simulink model "sysModel"  (R2017a)
settings: Solver=FixedStepDiscrete  StartTime=0.0  StopTime=10.0  FixedStep=0.1  RelTol=1e-3  EnableMultiTasking=on
settings Model: Creator=plima  LastModifiedBy=plima
settings SolverCC: AutoInsertRateTranBlk=on
settings DataIOCC: LimitDataPoints=on
settings OptimizationCC: LifeSpan=inf
settings DebuggingCC: AllowSymbolicDim=off  SFUnexpectedBacktrackingDiag=warning  SFNoUnconditionalDefaultTransitionDiag=warning  SFExecutionAtInitializationDiag=none
settings GRTTargetCC: TargetLangStandard=C89/C90 (ANSI)  GeneratePreprocessorConditionals=Disable all
settings ConfigComp: CovMetricSettings=dw  CovHtmlReporting=on  CovSaveCumulativeToWorkspaceVar=on  CovSaveSingleToWorkspaceVar=on  CovShowResultsExplorer=off  CovExternalEMLEnable=off  CovSFcnEnable=off

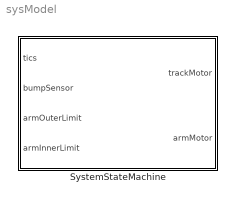
== system sysModel ==
  SystemStateMachine : Stateflow chart  TreatAsAtomicUnit=on

== stateflow chart sysModel/SystemStateMachine ==
  state ExtendArms
    entry: loopTics = tics;
    trackMotor = 0;
    during: armMotor = 1;
  state MoveOverBump
    during: armMotor = 0;
    trackMotor = 1;
  state RetractArms
    during: armMotor = -1;
  state BumpRetractArms
    during: armMotor = -1
  state MoveForward
    during: armMotor = 0;
    trackMotor = 1;
  state BumpExtendArms
    entry: loopTics = tics;
    trackMotor = 0;
    during: armMotor = 1
  state SystemStop
    during: armMotor = 0;
  state FinalRetractArms
    during: armMotor = -1;
  state FinalExtendArms
    entry: trackMotor = 0;
    during: armMotor = 1;
  (default) -> ExtendArms : /{initialTics = tics}
  MoveOverBump -> ExtendArms : [tics - loopTics >= VehicleLength + BumpLength]
  MoveForward -> ExtendArms [order 1] : [tics - loopTics >= VehicleLength]
  BumpRetractArms -> MoveOverBump : [armInnerLimit == 1]
  ExtendArms -> RetractArms : [armOuterLimit == 1]
  BumpExtendArms -> BumpRetractArms : [armOuterLimit == 1]
  RetractArms -> MoveForward : [armInnerLimit == 1]
  MoveForward -> BumpExtendArms [order 2] : [bumpSensor == 1]
  MoveForward -> FinalExtendArms [order 3] : [tics >= WindowLength + initialTics]
  FinalRetractArms -> SystemStop : [armInnerLimit == 1]
  FinalExtendArms -> FinalRetractArms : [armOuterLimit == 1]
  data: trackMotor output; tics input; bumpSensor input; armMotor output; armOuterLimit input; armInnerLimit input; VehicleLength constant double; loopTics local; WindowLength constant double; BumpLength constant double; initialTics local
